simulink model "Main_simulation_optimised_accel_testbed"  (R2017b)
settings: Solver=FixedStepDiscrete  StartTime=0  StopTime=2474  RelTol=1e-3  EnableMultiTasking=on
PreLoadFcn:
  | Ts=2e-6;
undefined symbols (not defined in the file): Batt, BatteryCback, BatteryLoadFcn, DiscIntNeverNeededParam, Discrete, gcbh, Ion, Lithium, sigbuilder_block, sps_rtmsupport, spsBatteryModel
libraries: powerlib x53, electricdrivelib x6, simulink x6, autolibshared x6, powerlib_meascontrol x4, sdolib x3, spsDrivesDcBusModel x1, spsDrivesPrivateModels x1, spsDrivesOutputSelector x1, spsDrivesSpeedControllerModel x1
(part 1 of 3)
Description:
  | Copyright 2008-2017 The MathWorks, Inc.
settings Model: SimulationMode=accelerator  ExtModeAutoUpdateStatusClock=off  Creator=MathWorks  LastModifiedBy=LENOVO
settings SolverCC: AlgebraicLoopSolver=LineSearch  AutoInsertRateTranBlk=on
settings DataIOCC: LimitDataPoints=on  SaveFormat=Array  SignalLoggingSaveFormat=ModelDataLogs  SaveOutput=off  SignalLogging=off  SaveTime=off  SignalLoggingName=sigsOut
settings OptimizationCC: ExpressionDepthLimit=2147483647  InitFltsAndDblsToZero=on  LifeSpan=inf
settings DebuggingCC: UnderspecifiedInitializationDetection=Classic  MergeDetectMultiDrivingBlocksExec=none  CheckExecutionContextPreStartOutputMsg=on  CheckExecutionContextRuntimeOutputMsg=on  SignalResolutionControl=TryResolveAllWithWarning  MultiTaskDSMMsg=warning  MultiTaskCondExecSysMsg=none  FcnCallInpInsideContextMsg=warning  StateNameClashWarn=warning  SFUnexpectedBacktrackingDiag=warning  SFNoUnconditionalDefaultTransitionDiag=warning  SFExecutionAtInitializationDiag=none
settings HardwareCC: ProdBitPerPointer=32  ProdBitPerSizeT=32  ProdBitPerPtrDiffT=32  ProdLargestAtomicFloat=None  ProdIntDivRoundTo=Undefined  ProdEndianess=Unspecified  ProdWordSize=32  ProdHWDeviceType=32-bit Generic  TargetUnknown=on
settings ModelReferenceCC: PropagateSignalLabelsOutOfModel=off
settings CodeAppCC: StateflowObjectComments=on
settings GRTTargetCC: TargetLangStandard=C89/C90 (ANSI)  GeneratePreprocessorConditionals=Disable all  CombineOutputUpdateFcns=off  GRTInterface=on
settings ConfigComp: CovMetricSettings=dw  CovHtmlReporting=on  CovSaveCumulativeToWorkspaceVar=on  CovSaveSingleToWorkspaceVar=on  CovExternalEMLEnable=off  CovSFcnEnable=off
settings SimscapeCC: SimscapeNormalizeSystem=off

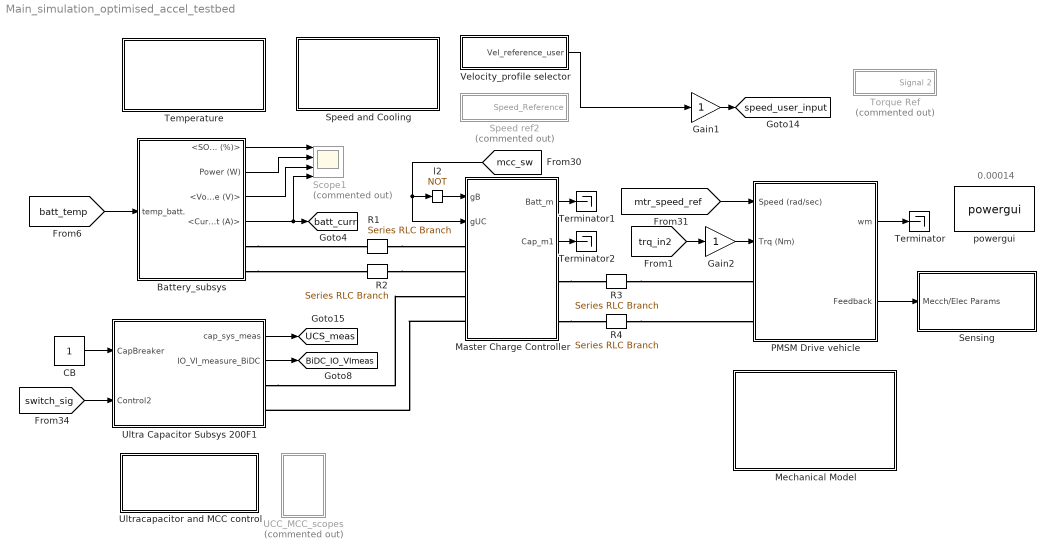
== system Main_simulation_optimised_accel_testbed ==
  note: 0.00014
  Battery_subsys : Subsystem
  CB : Constant
  Gain1 : Gain
  Gain2 : Gain
  Master Charge Controller : Subsystem
  Mechanical Model : Subsystem
  PMSM Drive vehicle : Subsystem
  R{1..4} (4 alike) : powerlib/Elements/Series RLC Branch  LConnTagsString=__new0  RConnTagsString=__new0  BranchType=R  Resistance=0.02  Inductance=220e-6  SetiL0=off  InitialCurrent=0  Capacitance=447e-6  Setx0=off  InitialVoltage=0  Measurements=None
  Scope1 : Scope  Commented=on  NumInputPorts=4
  Sensing : Subsystem
  "Speed and Cooling " : Subsystem
  Speed ref2 : Subsystem  Tag=STV Subsys  Commented=on  LoadFcn=sigbuilder_block('load');  StartFcn=sigbuilder_block('start');  StopFcn=sigbuilder_block('stop');  ClipboardFcn=sigbuilder_block('clipboard');  mask(Sigbuilder block){tuvar=[0:10]}
      mask help: Simulink:masks:SigbuilderBlock_MD
      mask init:
      | if ~strcmp(get_param(bdroot(gcbh),'SimulationStatus'),'stopped') tuvar = sigbuilder_block('maskInit'); end
      settings: CopyFcn=sigbuilder_block('copy');  DeleteFcn=sigbuilder_block('delete');  ModelCloseFcn=sigbuilder_block('modelClose');  PreSaveFcn=sigbuilder_block('preSave');  PauseFcn=sigbuilder_block('pause');  ContinueFcn=sigbuilder_block('continue');  NameChangeFcn=sigbuilder_block('namechange');  OpenFcn=sigbuilder_block('open',[5.4 30 1141.2 522.6 ]);  CloseFcn=sigbuilder_block('close');
      mask Display: plot(0, 0, 100, 100,[2, 2, 32, 32, 2], [68, 8, 8, 68, 68],[32, 2], [38, 38], [32, 19, 2],[53, 60, 44], [32, 17, 17, 2],[16, 16, 31, 31]);txt = getActiveGroup(gcbh);text(2, 100, txt,'verticalAlignment', 'top');
  Temperature : Subsystem
  Terminator : Terminator
  Terminator1 : Terminator
  Terminator2 : Terminator
  Torque Ref : Subsystem  Tag=STV Subsys  Commented=on  LoadFcn=sigbuilder_block('load');  StartFcn=sigbuilder_block('start');  StopFcn=sigbuilder_block('stop');  ClipboardFcn=sigbuilder_block('clipboard');  mask(Sigbuilder block){tuvar=[0:10]}
      mask help: Simulink:masks:SigbuilderBlock_MD
      mask init:
      | if ~strcmp(get_param(bdroot(gcbh),'SimulationStatus'),'stopped') tuvar = sigbuilder_block('maskInit'); end
      settings: CopyFcn=sigbuilder_block('copy');  DeleteFcn=sigbuilder_block('delete');  ModelCloseFcn=sigbuilder_block('modelClose');  PreSaveFcn=sigbuilder_block('preSave');  PauseFcn=sigbuilder_block('pause');  ContinueFcn=sigbuilder_block('continue');  NameChangeFcn=sigbuilder_block('namechange');  OpenFcn=sigbuilder_block('open',[5.4 30 1141.2 522.6 ]);  CloseFcn=sigbuilder_block('close');
      mask Display: plot(0, 0, 100, 100,[2, 2, 32, 32, 2], [68, 8, 8, 68, 68],[32, 2], [38, 38], [32, 19, 2],[53, 60, 44], [32, 17, 17, 2],[16, 16, 31, 31]);txt = getActiveGroup(gcbh);text(2, 100, txt,'verticalAlignment', 'top');
  "UCC_MCC_scopes " : Subsystem  Commented=on
  Ultra Capacitor Subsys 200F1 : Subsystem
  Ultracapacitor and MCC control : Subsystem
  Velocity_profile selector : Subsystem
  l2 : Logic  Operator=NOT  IconShape=distinctive  AllPortsSameDT=off  OutDataTypeStr=boolean
  powergui : powerlib/powergui  Priority=2  SimulationMode=Discrete  SampleTime=1e-6  frequency=60  Iterations=50  frequencyindice=0  Pbase=100e6  ErrMax=1e-4  UnitsV=kV  UnitsW=MW  buscounter=0  FunctionMessages=off  echomessages=off  EnableUseOfTLC=off  CurrentSourceSwitches=off  DisableSnubberDevices=off  DisableRonSwitches=off  DisableVfSwitches=off  DisplayEquations=off  SolverType=Tustin/Backward Euler (TBE)  Interpol=off  ExternalGateDelay=off  methode=off  Ts=0  x0status=blocks  SPID=off  SwTol=0  HookPort=off  RestoreLinks=warning  ResistiveCurrentMeasurement=off  Frange=[0:2:500]  Ylog=off  Xlog=on  ShowGrid=off  save=off  variable=ZData  structure=0  ZoomFFT=on  StartTime=0.0  cycles=1  DisplayStyle=1  fundamental=60  FreqAxis=off  MaxFrequency=1000  frequencyindicesteady=1  RmsSteady=1  display=off
  tag scope: BiDC_IO_VImeas=global, UCS_meas=global, batt_curr=global, speed_user_input=global
  wires:
  Velocity_profile selector/1(Vel_reference_user) -> Gain1/1
  [trq_in2] -> Gain2/1
  Gain2/1 -> PMSM Drive vehicle/2(Trq (Nm))
  PMSM Drive vehicle/1(wm) -> Terminator/1
  PMSM Drive vehicle/2(Feedback) -> Sensing/1(Mecch/Elec Params)
  Battery_subsys/4(<Current (A)>) -> Scope1/4, [batt_curr]
  [batt_temp] -> Battery_subsys/1(temp_batt.)
  Battery_subsys/2(Power (W)) -> Scope1/2
  Battery_subsys/1(<SOC (%)>) -> Scope1/1
  Battery_subsys/3(<Voltage (V)>) -> Scope1/3
  [mcc_sw] -> Master Charge Controller/2(gUC), l2/1
  CB/1 -> Ultra Capacitor Subsys 200F1/1(CapBreaker)
  Ultra Capacitor Subsys 200F1/1(cap_sys_meas) -> [UCS_meas]
  l2/1 -> Master Charge Controller/1(gB)
  [switch_sig] -> Ultra Capacitor Subsys 200F1/2(Control2)
  [mtr_speed_ref] -> PMSM Drive vehicle/1(Speed (rad/sec))
  Ultra Capacitor Subsys 200F1/2(IO_VI_measure_BiDC) -> [BiDC_IO_VImeas]
  Master Charge Controller/1(Batt_m) -> Terminator1/1
  Master Charge Controller/2(Cap_m1) -> Terminator2/1
  Gain1/1 -> [speed_user_input]
  connections:
  Master Charge Controller/RConn1 -- R3/RConn1
  Master Charge Controller/RConn2 -- R4/RConn1
  Battery_subsys/RConn1 -- R1/RConn1
  Battery_subsys/RConn2 -- R2/RConn1
  Ultra Capacitor Subsys 200F1/RConn1 -- Master Charge Controller/LConn3
  Master Charge Controller/LConn4 -- Ultra Capacitor Subsys 200F1/RConn2
  R1/LConn1 -- Master Charge Controller/LConn1
  R2/LConn1 -- Master Charge Controller/LConn2
  R3/LConn1 -- PMSM Drive vehicle/LConn1
  R4/LConn1 -- PMSM Drive vehicle/LConn2

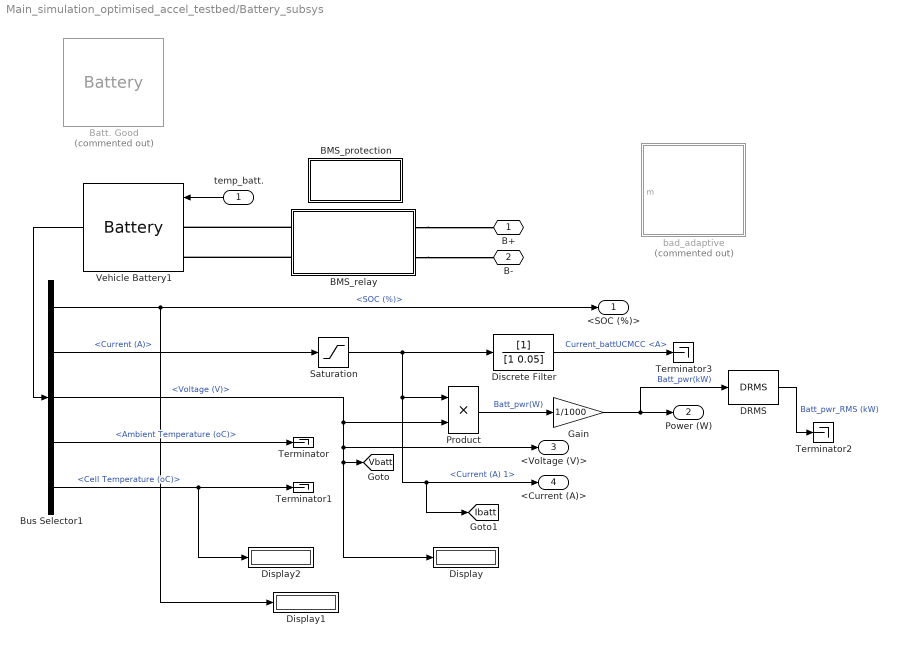
== system Main_simulation_optimised_accel_testbed/Battery_subsys ==
  temp_batt. : Inport
  BMS_protection : Subsystem
  BMS_relay : Subsystem
  Batt. Good : electricdrivelib/Extra Sources/Battery  Commented=on  BatType=Lithium-Ion  ShowTempParam=on  ThermalPreset=no  ShowAgeParam=off  NomV=120  NomQ=66  SOC=96  Batt_Tr=0.1  PresetModel=off  MaxQ=66  MinV=90  FullV=130  Dis_rate=30  R=0.018182  Normal_OP=59.687  expZone="[129.6463      3.242609]"  current=[6.5 13 18 22 32.5 40]  Units=Time  Tci=20  NomT=50  T2=-15  MaxQ2=60*0.7  FullV2=117  Normal_OP2=120*0.9  expZone2="[120        50]"  Rca=0.5  ti=1  Dp=0  Neq0=1  Tsim=50e-6  Ta1=35  Qeol=60*0.85  Reol=0.013333*1.2  Char_age=[2.3478, 3]  Dis_age=[2.3478, 10]  N1=1500  N2=10500  N3=1000  N4=1400  Ta2=45  N5=950
  Bus Selector1 : BusSelector  OutputSignals=SOC (%),Current (A),Voltage (V),Ambient Temperature (oC),Cell Temperature (oC)
  DRMS : sdolib/RMS Blocks/DRMS  Ts=10e-6
      settings: SourceProductName=Simulink Design Optimization  SourceProductBaseCode=SO
  Discrete Filter : DiscreteFilter  Denominator=[1 0.05]
  Display : Display
  Display1 : Display
  Display2 : Display
  Gain : Gain  Gain=1/1000
  Product : Product
  Saturation : Saturate  UpperLimit=50  LowerLimit=-40
  Terminator{,1..3} (4 alike) : Terminator
  Vehicle Battery1 : electricdrivelib/Extra Sources/Battery  BatType=Lithium-Ion  ShowTempParam=on  ThermalPreset=no  ShowAgeParam=off  NomV=120  NomQ=66  SOC=30  Batt_Tr=0.1  PresetModel=off  MaxQ=66  MinV=90  FullV=130  Dis_rate=30  R=0.018182  Normal_OP=59.687  expZone="[129.6463      3.242609]"  current=[6.5 13 18 22 32.5 40]  Units=Time  Tci=20  NomT=50  T2=-15  MaxQ2=60*0.7  FullV2=117  Normal_OP2=120*0.9  expZone2="[120        50]"  Rca=0.5  ti=1  Dp=0  Neq0=1  Tsim=50e-6  Ta1=35  Qeol=60*0.85  Reol=0.013333*1.2  Char_age=[2.3478, 3]  Dis_age=[2.3478, 10]  N1=1500  N2=10500  N3=1000  N4=1400  Ta2=45  N5=950
  bad_adaptive : Subsystem  Commented=on  DialogController=POWERSYS.PowerSysDialog  LoadFcn=sps_rtmsupport('LoadFcn',gcbh); BatteryLoadFcn(gcb)  InitFcn=BatteryCback(gcb,1)  StartFcn=sps_rtmsupport('StartFcn',gcbh);  StopFcn=sps_rtmsupport('StopFcn',gcbh);  mask(Battery){BatType=Lithium-Ion, ShowTempParam=off, ThermalPreset=no, ShowAgeParam=off, NomV=120, NomQ=66, SOC=96, Batt_Tr=0.1, PresetModel=off, MaxQ=66, MinV=90, FullV=130, Dis_rate=30, R=0.018182, Normal_OP=59.687, expZone=[129.6463      3.242609], current=[6.5 13 18 22 32.5 40], Units=Time, Tci=20, NomT=50, T2=-15, MaxQ2=60*0.7, FullV2=117, Normal_OP2=120*0.9, expZone2=[120        50], Rca=0.5, ti=1, Dp=0, Neq0=1, Tsim=50e-6, Ta1=35, Qeol=60*0.85, Reol=0.013333*1.2, Char_age=[2.3478, 3], Dis_age=[2.3478, 10], N1=1500, N2=10500, N3=1000, N4=1400, Ta2=45, N5=950}
      mask prompts: BatType "Type:"; ShowTempParam "Simulate temperature effects"; ThermalPreset "Use a preset battery:"; ShowAgeParam "Simulate aging effects"; NomV "Nominal voltage (V)"; NomQ "Rated capacity (Ah)"; SOC "Initial state-of-charge (%)"; Batt_Tr "Battery response time (s)"; PresetModel "Determined from the nominal parameters of the battery"; MaxQ "Maximum capacity (Ah)"; MinV "Cut-off Voltage (V)"; FullV "Fully charged voltage (V)"; Dis_rate "Nominal discharge current (A)"; R "Internal resistance (Ohms)"; Normal_OP "Capacity (Ah) at nominal voltage"; expZone "Exponential zone [Voltage (V), Capacity (Ah)]"; current "Discharge current [i1, i2, i3,...] (A)"; Tci "Initial cell temperature (deg. C)"; NomT "Nominal ambient temperature T1 (deg. C)"; T2 "Second ambient temperature T2 (deg. C)"; MaxQ2 "Maximum capacity (Ah)"; FullV2 "Initial discharge voltage (V)"; Normal_OP2 "Voltage at 90% maximum capacity (V)"; expZone2 "Exponential zone [Voltage (V), Capacity (Ah)]"; Rca "Thermal resistance, cell-to-ambient (deg. C/W)"; ti "Thermal time constant, cell-to-ambient (s)"; Dp "Heat loss difference [charge vs. discharge] (W)"; Neq0 "Initial battery age (Equivalent full cycles)"; Tsim "Aging model sampling time (s)"; Ta1 "Ambient temperature Ta1 (deg. C)"; Qeol "Capacity at EOL (End Of Life) (Ah)"; Reol "Internal resistance at EOL (Ohms)"; Char_age "Charge current (nominal, maximum) [Ic (A), Icmax (A)]"; Dis_age "Discharge current (nominal, maximum) [Id (A), Idmax (A)]"; N1 "Cycle life at 100 % DOD, Ic and Id (Cycles)"; N2 "Cycle life at 25 % DOD, Ic and Id (Cycles)"; N3 "Cycle life at 100 % DOD, Ic and Idmax (Cycles)"; N4 "Cycle life at 100 % DOD, Icmax and Id (Cycles)"; Ta2 "Ambient temperature Ta2 (deg. C)"; N5 "Cycle life at 100 % DOD, Ic and Id (Cycles)"
      mask help: Implements a generic battery model for most popular battery types. Temperature and aging (due to cycling) effects can be specified for Lithium-Ion battery type.
      mask init:
      | block = gcb;
      | BatteryCback(block,3)
      | [Batt BT, WantBlockChoice, Ts] = BatteryParam(NomV,NomQ,MaxQ,MinV,FullV,Dis_rate,R,Normal_OP,expZone,block,0);
      | powericon('SetInternalModels','set',block,WantBlockChoice);
      | BatteryCback(block,1);
      settings: CopyFcn=sps_rtmsupport('CopyFcn',gcbh);  DeleteFcn=sps_rtmsupport('DeleteFcn',gcbh);  UndoDeleteFcn=sps_rtmsupport('UndoDeleteFcn',gcbh);  ModelCloseFcn=sps_rtmsupport('ModelCloseFcn',gcbh);  PreSaveFcn=sps_rtmsupport('PreSaveFcn',gcbh);  PostSaveFcn=sps_rtmsupport('PostSaveFcn',gcbh);  NameChangeFcn=sps_rtmsupport('NameChangeFcn',gcbh);  PreCopyFcn=sps_rtmsupport('PreCopyFcn',gcbh);  OpenFcn=sps_rtmsupport('OpenFcn',gcbh, [1,2,3,4,9,18]);  CloseFcn=sps_rtmsupport('CloseFcn',gcbh);  PreDeleteFcn=sps_rtmsupport('PreDeleteFcn',gcbh);
      mask Help: helpview(psbhelp)
      mask TypeOptions BatType: Lead-Acid | Lithium-Ion | Nickel-Cadmium | Nickel-Metal-Hydride
      mask Callback BatType: BatteryCback(gcb,1)
      mask Callback ShowTempParam: BatteryCback(gcb,1)
      mask TypeOptions ThermalPreset: no | 3.3V  2.3Ah  (LiFePO4) | 3.6V  2050mAh   (LiCoO2) | 3.6V  2.0Ah | 3.6V  3.6Ah  (LiNiO2) | 3.6V  4.5Ah | 3.6V  48Ah  (LiNiO2) | 3.7V  4.4Ah | 7.4V  5.4Ah  (LiCoO2) | 11.1V  6600mAh  (LiCoO2) | 12.8V  40Ah  (LiFeMgPO4)
      mask Callback ThermalPreset: BatteryCback(gcb,4)
      mask Callback ShowAgeParam: BatteryCback(gcb,1)
      mask Callback PresetModel: BatteryCback(gcb,1)
      mask TypeOptions Units: Ampere-hour | Time
      mask Callback ti: sps_rtmsupport('parametereditingmodes',gcbh, [1,2,3,4,9,18]);
      mask DialogControl ParameterTabVar0 Prompt: Parameters
      mask DialogControl Tempcontainer Prompt: Temperature
      mask DialogControl Agecontainer Prompt: Aging
      mask DialogControl ParameterTabVar01 Prompt: Discharge
      mask DialogControl Container9 Prompt: Display characteristics
      mask DialogControl PlotButton Prompt: Plot
      mask DialogControl PlotButton Callback: BatteryCback(gcb,0)
      mask DialogControl Temperature Prompt: Temperature
      mask DialogControl Container7 Prompt: Discharge parameters at T2
      mask DialogControl Container8 Prompt: Thermal response and Heat loss
      mask DialogControl Aging Prompt: Aging
      mask DialogControl Container16 Prompt: Aging characteristics at ambient temperature Ta1
      mask DialogControl Container13 Prompt: Aging characteristics at ambient temperature Ta2
      mask Display:
      | patch([BT.X1 BT.X1m],[BT.Y1 BT.Y1m],BT.color1);
      | patch(BT.X3,BT.Y3,BT.color2);
      | plot([BT.X1 BT.X1m BT.X2 BT.X2m BT.X3 BT.X4],[BT.Y1 BT.Y1m BT.Y2 BT.Y2m BT.Y3 BT.Y4]);
      | plot(-100,-60,60,50,[BT.X(1) BT.X(1)],[BT.bas BT.haut],[BT.X(2) BT.X(2)],[BT.haut BT.bas],BT.dim_Xsin,4*sin(BT.dim_sin)+BT.haut,BT.dim_Xsin,-4*sin(BT.dim_sin)+BT.haut,BT.dim_Xsin,-4*sin(BT.dim_sin)+BT.bas,BT.dim_Xtop,sin(BT.dim_top)+BT.haut+4,BT.dim_Xtop,-sin(BT.dim_top)+BT.haut+4,BT.dim_Xtop,-sin(BT.dim_top)+BT.haut,[BT.TopX(2),BT.TopX(2)],[BT.haut,BT.haut+4],[BT.TopX(1),BT.TopX(1)],[BT.haut+4,BT.haut]);plot(BT.dim_Xsin,-5*sin(BT.dim_sin)+20);
      | port_label('lconn',1,'+');
      | port_label('lconn',2,'_');
      | color('blue');
      | port_label('output',1,'m');
      | 
      | if Batt.sel_T
      |     port_label('input',1,'Ta');
      | end
  B+ : PMIOPort  Port=1  Side=Right
  B- : PMIOPort  Port=2  Side=Right
  <SOC (%)> : Outport
  Power (W) : Outport  Port=2
  <Voltage (V)> : Outport  Port=3
  <Current (A)> : Outport  Port=4
  tag scope: Ibatt=global, Vbatt=global
  wires:
  temp_batt./1 -> Vehicle Battery1/1
  Bus Selector1/2 -> Saturation/1  "<Current (A)>"
  Bus Selector1/1 -> Display1/1, <SOC (%)>/1  "<SOC (%)>"
  Product/1 -> Gain/1  "Batt_pwr(W)"
  Vehicle Battery1/1 -> Bus Selector1/1
  Bus Selector1/3 -> Product/2, <Voltage (V)>/1, Display/1, [Vbatt]  "<Voltage (V)>"
  Gain/1 -> Power (W)/1, DRMS/1  "Batt_pwr(kW)"
  Saturation/1 -> Product/1, <Current (A)>/1, [Ibatt], Discrete Filter/1  "<Current (A) 1>"
  Bus Selector1/4 -> Terminator/1  "<Ambient Temperature (oC)>"
  Bus Selector1/5 -> Display2/1, Terminator1/1  "<Cell Temperature (oC)>"
  DRMS/1 -> Terminator2/1  "Batt_pwr_RMS (kW)"
  Discrete Filter/1 -> Terminator3/1  "Current_battUCMCC <A>"
  connections:
  BMS_relay/LConn1 -- Vehicle Battery1/LConn1
  BMS_relay/LConn2 -- Vehicle Battery1/LConn2
  BMS_relay/RConn1 -- B+/RConn1
  BMS_relay/RConn2 -- B-/RConn1

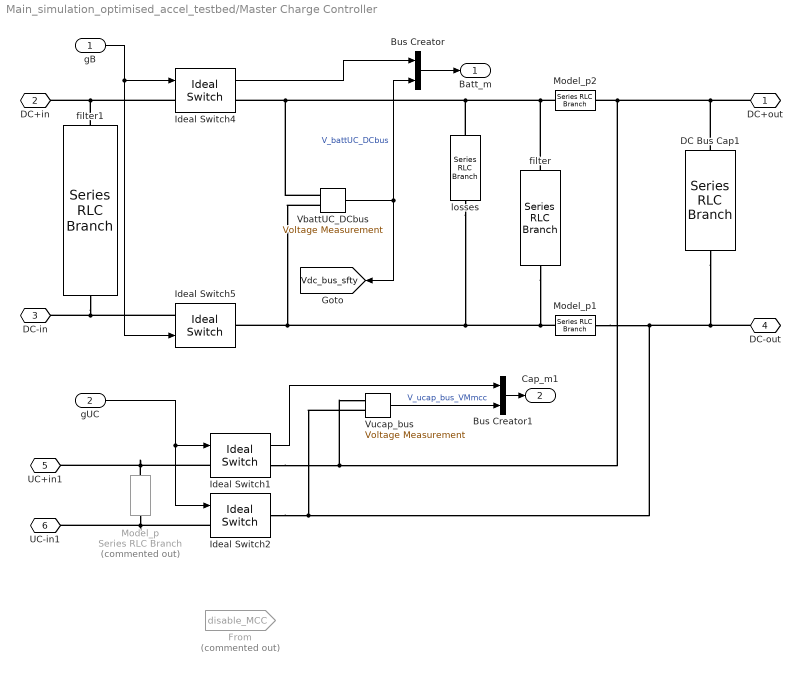
== system Main_simulation_optimised_accel_testbed/Master Charge Controller ==
  gB : Inport
  gUC : Inport  Port=2
  Bus Creator : BusCreator  Inputs=2
  Bus Creator1 : BusCreator  Inputs=2
  DC Bus Cap1 : powerlib/Elements/Series RLC Branch  LConnTagsString=__new0  RConnTagsString=__new0  BranchType=RC  Resistance=1e-2  Inductance=1e-3  SetiL0=off  InitialCurrent=0  Capacitance=400e-6  Setx0=off  InitialVoltage=0  Measurements=None
  From : From  Commented=on  GotoTag=disable_MCC  TagVisibility=global
  Ideal Switch1 : powerlib/Power Electronics/Ideal Switch  Ron=0.001  Lon=0  IC=0  Rs=1e6  Cs=10e-6  Measurements=on
  Ideal Switch2 : powerlib/Power Electronics/Ideal Switch  Ron=0.001  Lon=0  IC=0  Rs=1e6  Cs=10e-6  Measurements=off
  Ideal Switch4 : powerlib/Power Electronics/Ideal Switch  Ron=0.001  Lon=0  IC=0  Rs=10e6  Cs=10e-6  Measurements=on
  Ideal Switch5 : powerlib/Power Electronics/Ideal Switch  Ron=0.001  Lon=0  IC=0  Rs=10e6  Cs=10e-6  Measurements=off
  Model_p : powerlib/Elements/Series RLC Branch  Commented=on  LConnTagsString=__new0  RConnTagsString=__new0  BranchType=R  Resistance=10e6  Inductance=1e-3  SetiL0=off  InitialCurrent=0  Capacitance=0  Setx0=off  InitialVoltage=0  Measurements=None
  Model_p1 : powerlib/Elements/Series RLC Branch  LConnTagsString=__new0  RConnTagsString=__new0  BranchType=RL  Resistance=0.01  Inductance=20e-6  SetiL0=off  InitialCurrent=0  Capacitance=0  Setx0=off  InitialVoltage=0  Measurements=None
  Model_p2 : powerlib/Elements/Series RLC Branch  LConnTagsString=__new0  RConnTagsString=__new0  BranchType=RL  Resistance=0.01  Inductance=20e-6  SetiL0=off  InitialCurrent=0  Capacitance=0  Setx0=off  InitialVoltage=0  Measurements=None
  VbattUC_DCbus : powerlib/Measurements/Voltage Measurement  PhasorSimulation=off  OutputType=Complex  PSBequivalent=0
  Vucap_bus : powerlib/Measurements/Voltage Measurement  PhasorSimulation=off  OutputType=Complex  PSBequivalent=0
  filter : powerlib/Elements/Series RLC Branch  LConnTagsString=__new0  RConnTagsString=__new0  BranchType=RC  Resistance=1e-3  Inductance=1e-3  SetiL0=off  InitialCurrent=0  Capacitance=1e-6  Setx0=off  InitialVoltage=0  Measurements=None
  filter1 : powerlib/Elements/Series RLC Branch  LConnTagsString=__new0  RConnTagsString=__new0  BranchType=RC  Resistance=1e-3  Inductance=1e-3  SetiL0=off  InitialCurrent=0  Capacitance=1e-6  Setx0=off  InitialVoltage=0  Measurements=None
  losses : powerlib/Elements/Series RLC Branch  LConnTagsString=__new0  RConnTagsString=__new0  BranchType=R  Resistance=10e6  Inductance=1e-3  SetiL0=off  InitialCurrent=0  Capacitance=1e-6  Setx0=off  InitialVoltage=0  Measurements=None
  DC+out : PMIOPort  Port=1  Side=Right
  DC+in : PMIOPort  Port=2  Side=Left
  DC-in : PMIOPort  Port=3  Side=Left
  DC-out : PMIOPort  Port=4  Side=Right
  UC+in1 : PMIOPort  Port=5  Side=Left
  UC-in1 : PMIOPort  Port=6  Side=Left
  Batt_m : Outport
  Cap_m1 : Outport  Port=2
  tag scope: Vdc_bus_sfty=global
  wires:
  gB/1 -> Ideal Switch5/1, Ideal Switch4/1
  Ideal Switch4/1 -> Bus Creator/1
  Ideal Switch1/1 -> Bus Creator1/1
  gUC/1 -> Ideal Switch2/1, Ideal Switch1/1
  VbattUC_DCbus/1 -> [Vdc_bus_sfty], Bus Creator/2  "V_battUC_DCbus"
  Bus Creator/1 -> Batt_m/1
  Bus Creator1/1 -> Cap_m1/1
  Vucap_bus/1 -> Bus Creator1/2  "V_ucap_bus_VMmcc"
  connections:
  Vucap_bus/LConn2 -- Ideal Switch2/RConn1 -- DC-out/RConn1 -- DC Bus Cap1/RConn1 -- Model_p1/LConn1
  Vucap_bus/LConn1 -- Ideal Switch1/RConn1 -- DC+out/RConn1 -- DC Bus Cap1/LConn1 -- Model_p2/LConn1
  Ideal Switch4/LConn1 -- filter1/LConn1 -- DC+in/RConn1
  Ideal Switch5/LConn1 -- filter1/RConn1 -- DC-in/RConn1
  Ideal Switch1/LConn1 -- Model_p/LConn1 -- UC+in1/RConn1
  Ideal Switch2/LConn1 -- Model_p/RConn1 -- UC-in1/RConn1
  losses/RConn1 -- VbattUC_DCbus/LConn2 -- Ideal Switch5/RConn1 -- Model_p1/RConn1 -- filter/RConn1
  losses/LConn1 -- Model_p2/RConn1 -- filter/LConn1 -- VbattUC_DCbus/LConn1 -- Ideal Switch4/RConn1

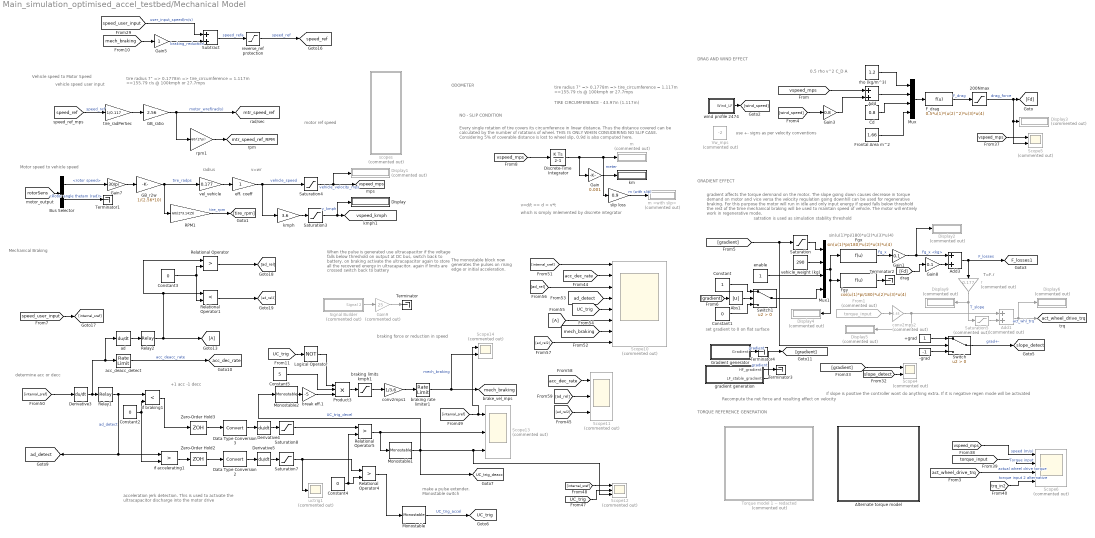
== system Main_simulation_optimised_accel_testbed/Mechanical Model ==
  note: sin(u(1)*pi/180)*u(2)*u(3)*u(4)
  note: set gradient to 0 on flat surface
  note: Recompute the net force and resulting effect on velocity
  note: Vehicle speed to Motor Speed
  note: motor ref speed
  note: tire radius 7" => 0.1778m => tire_circumference = 1.117m
      | =>155.79 r/s @ 100kmph or 27.7mps
  note: vehicle speed
      | user input
  note: v=wr
  note: Motor speed to vehicle speed
  note: radius
  note: T=F.r
  note: use +- signs as per velocity conventions
  note: satration is used as simulation stability threshold
  note: gradient affects the torque demnand on the motor. The slope going down causes decrease in torque demand on motor and vice versa
      |
      | the velocity regulation going downhill can be used for regenerative braking. For this purpose the motor will run in idle and only input energy if speed falls below threshold
      | the rest of the time mechanical braking will be used to maintain speed of vehicle. The motor will entirely work in regenerative mode.
  note: if slope is positive the controller wont do anything extra. If it is negative regen mode will be activated
  note: 0.5 rho v^2 C_D A
  note: GRADIENT EFFECT
  note: DRAG AND WIND EFFECT
  note: TORQUE REFERENCE GENERATION
  note: make a pulse extender.
      | Monostable switch
  note: acceleration jerk detection. This is used to activate the ultracapacitor discharge into the motor drive
  note: When the pulse is generated use ultracapacitor
      | if the voltage falls below threshold on output
      | at DC bus, switch back to battery.
      |
      | on braking activate the ultracapacitor again to store all
      | the recovered energy in ultracapacitor. again if limits are
      | crossed switch back to battery
  note: The monostable block
      | now generates the
      | pulses on rising edge or
      | initial acceleration.
  note: Mechanical Braking
  note: braking force or reduction in speed
  note: determine acc or decc
  note: +1 acc
      |  -1 decc
  note: NO - SLIP CONDITION
  note: which is simply imlemented by discrete integrator
  note: v=d/t => d = v*t
  note: ODOMETER
  note: Every single rotation of tire covers its circumference in linear distance. Thus the distance covered
      | can be calculated by the number of rotations of wheel. THIS IS ONLY WHEN CONSIDERING
      | NO SLIP CASE. Considering 5% of coverable distance is lost to wheel slip, 0.9d is also computed here.
  note: TIRE CIRCUMFERENCE - 43.97in (1.117m)
  note: tire radius 7" => 0.1778m => tire_circumference = 1.117m
      | =>155.79 r/s @ 100kmph or 27.7mps
  +grad : Constant
  -grad : Constant  Value=-1
  200Nmax : Saturate  UpperLimit=200  LowerLimit=0
  Abs1 : Abs
  Add : Sum
  Add1 : Sum  Commented=on
  Add3 : Sum
  Alternate torque model : Subsystem
  Bus Selector : BusSelector  OutputSignals=rotor speed,Rotor angle thetam (rad)
  Cd : Constant  Value=0.8
  Constant : Constant
  Constant{1..4} (4 alike) : Constant  Value=0
  Constant5 : Constant  Value=5
  Data Type Conversion2 : DataTypeConversion
  Data Type Conversion3 : DataTypeConversion
  Derivative3 : Derivative
  Derivative4 : Derivative
  Derivative5 : Derivative
  Discrete-Time Integrator : DiscreteIntegrator  InitialConditionSetting=State (most efficient)  SampleTime=-1  ICPrevOutput=DiscIntNeverNeededParam  ICPrevScaledInput=DiscIntNeverNeededParam
  Display : Display
  Display{1..6,9} (7 alike) : Display  Commented=on
  F_drag : Fcn  Expr=0.5*u(1)*(u(2)^2)*u(3)*u(4)
  Fgx : Fcn  Expr=sin(u(1)*pi/180)*u(2)*u(3)*u(4)
  Fgy : Fcn  Expr=cos(u(1)*pi/180)*u(2)*u(3)*u(4)
  From1 : From  Commented=on  GotoTag=torque_input  TagVisibility=global
  Frontal Area m^2 : Constant  Value=1.66
  GB_r2w : Gain  Gain=1/(2.56*10)
  GB_ratio : Gain  Gain=2.56
  Gain : Gain  Gain=0.001
  Gain1 : Gain  Gain=0.1
  Gain3 : Gain  Gain=0.8
  Gain5 : Gain
  Gain7 : Gain  Gain=30/pi  SaturateOnIntegerOverflow=on  OutDataTypeStr=Inherit: Same as input  ParamDataTypeStr=Inherit: Same as input
  Gain8 : Gain  Gain=0.1
  Gain9 : Gain  Commented=on  Gain=25
  Gradient generator : Subsystem  Tag=STV Subsys  LoadFcn=sigbuilder_block('load');  StartFcn=sigbuilder_block('start');  StopFcn=sigbuilder_block('stop');  ClipboardFcn=sigbuilder_block('clipboard');  mask(Sigbuilder block){tuvar=[0:10]}
      mask help: Simulink:masks:SigbuilderBlock_MD
      mask init:
      | if ~strcmp(get_param(bdroot(gcbh),'SimulationStatus'),'stopped') tuvar = sigbuilder_block('maskInit'); end
      settings: CopyFcn=sigbuilder_block('copy');  DeleteFcn=sigbuilder_block('delete');  ModelCloseFcn=sigbuilder_block('modelClose');  PreSaveFcn=sigbuilder_block('preSave');  PauseFcn=sigbuilder_block('pause');  ContinueFcn=sigbuilder_block('continue');  NameChangeFcn=sigbuilder_block('namechange');  OpenFcn=sigbuilder_block('open',[0 30 1152 561.6 ]);  CloseFcn=sigbuilder_block('close');
      mask Display: plot(0, 0, 100, 100,[2, 2, 32, 32, 2], [68, 8, 8, 68, 68],[32, 2], [38, 38], [32, 19, 2],[53, 60, 44], [32, 17, 17, 2],[16, 16, 31, 31]);txt = getActiveGroup(gcbh);text(2, 100, txt,'verticalAlignment', 'top');
  Logical Operator : Logic  Operator=NOT  IconShape=distinctive  AllPortsSameDT=off  OutDataTypeStr=boolean
  Monostable : powerlib_meascontrol/Logic/Monostable  EdgeDetect=Rising  PulseDuration=0.4  ic=0  Ts=0
      settings: SourceProductName=Simscape Power Systems  SourceProductBaseCode=PS
  Monostable1 : powerlib_meascontrol/Logic/Monostable  EdgeDetect=Rising  PulseDuration=0.15  ic=0  Ts=0
      settings: SourceProductName=Simscape Power Systems  SourceProductBaseCode=PS
  Monostable2 : powerlib_meascontrol/Logic/Monostable  EdgeDetect=Rising  PulseDuration=0.45  ic=0  Ts=0
      settings: SourceProductName=Simscape Power Systems  SourceProductBaseCode=PS
  Mux : Mux
  Mux1 : Mux
  Product3 : Product  Inputs=3
  RPM1 : Gain  Gain=60/(2*3.1415)
  Relational Operator : RelationalOperator  Operator=>  OutDataTypeStr=boolean  RndMeth=Simplest
  Relational Operator1 : RelationalOperator  Operator=<  OutDataTypeStr=boolean  RndMeth=Simplest
  Relational Operator4 : RelationalOperator  Operator=>  OutDataTypeStr=boolean  RndMeth=Simplest
  Relational Operator5 : RelationalOperator  Operator=>  OutDataTypeStr=boolean  RndMeth=Simplest
  Relay1 : Relay  OffOutputValue=-1
  Relay2 : Relay  OffOutputValue=-1
  Saturation : Saturate  UpperLimit=10  LowerLimit=-10
  Saturation3 : Saturate  UpperLimit=108  LowerLimit=0
  Saturation4 : Saturate  UpperLimit=30  LowerLimit=0
  Saturation5 : Saturate  Commented=on  UpperLimit=25  LowerLimit=-25
  Saturation7 : Saturate  UpperLimit=10  LowerLimit=-10
  Saturation8 : Saturate  UpperLimit=10  LowerLimit=-10
  Scope10 : Scope  Commented=on  NumInputPorts=8
  Scope11 : Scope  Commented=on  NumInputPorts=3
  Scope12 : Scope  Commented=on  NumInputPorts=3
  Scope13 : Scope  Commented=on  NumInputPorts=3
  Scope14 : Scope  Commented=on  NumInputPorts=2
  Scope4 : Scope  Commented=on  NumInputPorts=2
  Scope5 : Scope  Commented=on  NumInputPorts=2
  Scope6 : Scope  Commented=on  NumInputPorts=4
  Signal Builder : Subsystem  Tag=STV Subsys  Commented=on  LoadFcn=sigbuilder_block('load');  StartFcn=sigbuilder_block('start');  StopFcn=sigbuilder_block('stop');  ClipboardFcn=sigbuilder_block('clipboard');  mask(Sigbuilder block){tuvar=[0:10]}
      mask help: Simulink:masks:SigbuilderBlock_MD
      mask init:
      | if ~strcmp(get_param(bdroot(gcbh),'SimulationStatus'),'stopped') tuvar = sigbuilder_block('maskInit'); end
      settings: CopyFcn=sigbuilder_block('copy');  DeleteFcn=sigbuilder_block('delete');  ModelCloseFcn=sigbuilder_block('modelClose');  PreSaveFcn=sigbuilder_block('preSave');  PauseFcn=sigbuilder_block('pause');  ContinueFcn=sigbuilder_block('continue');  NameChangeFcn=sigbuilder_block('namechange');  OpenFcn=sigbuilder_block('open',[5.4 30 1141.2 522.6 ]);  CloseFcn=sigbuilder_block('close');
      mask Display: plot(0, 0, 100, 100,[2, 2, 32, 32, 2], [68, 8, 8, 68, 68],[32, 2], [38, 38], [32, 19, 2],[53, 60, 44], [32, 17, 17, 2],[16, 16, 31, 31]);txt = getActiveGroup(gcbh);text(2, 100, txt,'verticalAlignment', 'top');
  Subtract : Sum
  Switch : Switch  Criteria=u2 > Threshold
  Switch1 : Switch  Criteria=u2 > Threshold
  Terminator{,1..4} (5 alike) : Terminator
  "Torque model 1 -- redacted" : Subsystem  Commented=on
  Vw_mps : Constant  Commented=on  Value=-2
  Zero-Order Hold2 : ZeroOrderHold  SampleTime=-1
  Zero-Order Hold3 : ZeroOrderHold  SampleTime=-1
  acc_deacc_detect : RateLimiter  RisingSlewLimit=1000  FallingSlewLimit=-10e5  SampleTimeMode=inherited
  ad : Derivative
  braking limits kmph1 : Saturate  UpperLimit=0  LowerLimit=-40
  braking rate limiter1 : RateLimiter  RisingSlewLimit=10  FallingSlewLimit=-100  SampleTimeMode=inherited
  break eff.1 : Gain  Gain=-5
  conv2mps1 : Gain  Gain=1/3.6
  conv2mps2 : Gain  Commented=on  Gain=1.65
  eff. coeff : Gain
  enable : Constant
  gradient generation : Subsystem  Tag=STV Subsys  LoadFcn=sigbuilder_block('load');  StartFcn=sigbuilder_block('start');  StopFcn=sigbuilder_block('stop');  ClipboardFcn=sigbuilder_block('clipboard');  mask(Sigbuilder block){tuvar=[0:10]}
      mask help: Simulink:masks:SigbuilderBlock_MD
      mask init:
      | if ~strcmp(get_param(bdroot(gcbh),'SimulationStatus'),'stopped') tuvar = sigbuilder_block('maskInit'); end
      settings: CopyFcn=sigbuilder_block('copy');  DeleteFcn=sigbuilder_block('delete');  ModelCloseFcn=sigbuilder_block('modelClose');  PreSaveFcn=sigbuilder_block('preSave');  PauseFcn=sigbuilder_block('pause');  ContinueFcn=sigbuilder_block('continue');  NameChangeFcn=sigbuilder_block('namechange');  OpenFcn=sigbuilder_block('open',[5.4 30 1141.2 522.6 ]);  CloseFcn=sigbuilder_block('close');
      mask Display: plot(0, 0, 100, 100,[2, 2, 32, 32, 2], [68, 8, 8, 68, 68],[32, 2], [38, 38], [32, 19, 2],[53, 60, 44], [32, 17, 17, 2],[16, 16, 31, 31]);txt = getActiveGroup(gcbh);text(2, 100, txt,'verticalAlignment', 'top');
  if accelerating1 : RelationalOperator  Operator=>  OutDataTypeStr=boolean  RndMeth=Simplest
  if braking1 : RelationalOperator  Operator=<  OutDataTypeStr=boolean  RndMeth=Simplest
  km : Display
  kmph : Gain  Gain=3.6
  m : Display  Commented=on
  m <with slip> : Display  Commented=on
  r : Gain  Commented=on  Gain=0.177
  reverse_ref protection : Saturate  UpperLimit=45  LowerLimit=0
  rho (kg/m^3) : Constant  Value=1.2
  rpm1 : Gain  Gain=60/(2*pi)
  scopes : Subsystem  Commented=on
  slip loss : Gain  Gain=0.9
  tire_radPerSec : Gain  Gain=1/0.117
  uctrig1 : Scope  Commented=on
  vehicle_weight (kg) : Constant  Value=290
  vel_vehicle : Gain  Gain=0.177
  wind profile 2474 : Subsystem  Tag=STV Subsys  LoadFcn=sigbuilder_block('load');  StartFcn=sigbuilder_block('start');  StopFcn=sigbuilder_block('stop');  ClipboardFcn=sigbuilder_block('clipboard');  mask(Sigbuilder block){tuvar=[0:10]}
      mask help: Simulink:masks:SigbuilderBlock_MD
      mask init:
      | if ~strcmp(get_param(bdroot(gcbh),'SimulationStatus'),'stopped') tuvar = sigbuilder_block('maskInit'); end
      settings: CopyFcn=sigbuilder_block('copy');  DeleteFcn=sigbuilder_block('delete');  ModelCloseFcn=sigbuilder_block('modelClose');  PreSaveFcn=sigbuilder_block('preSave');  PauseFcn=sigbuilder_block('pause');  ContinueFcn=sigbuilder_block('continue');  NameChangeFcn=sigbuilder_block('namechange');  OpenFcn=sigbuilder_block('open',[5.4 30 1141.2 522.6 ]);  CloseFcn=sigbuilder_block('close');
      mask Display: plot(0, 0, 100, 100,[2, 2, 32, 32, 2], [68, 8, 8, 68, 68],[32, 2], [38, 38], [32, 19, 2],[53, 60, 44], [32, 17, 17, 2],[16, 16, 31, 31]);txt = getActiveGroup(gcbh);text(2, 100, txt,'verticalAlignment', 'top');
  tag scope: F_losses1=global, UC_trig=global, UC_trig_deacc=global, acc_dec_rate=global, act_wheel_drive_trq=global, ad_detect=global, mech_braking=global, mtr_speed_ref=global, mtr_speed_ref_RPM=global, slope_detect=global, speed_ref=global, vspeed_kmph=global, vspeed_mps=global
  wires:
  GB_ratio/1 -> rpm1/1, [mtr_speed_ref]  "motor_wref(rad/s)"
  Bus Selector/1 -> Gain7/1  "<rotor speed>"
  Bus Selector/2 -> Terminator1/1  "<Rotor angle thetam (rad)>"
  vel_vehicle/1 -> eff. coeff/1
  RPM1/1 -> [tire_rpm]  "tire_rpm"
  kmph/1 -> Saturation3/1
  Gain3/1 -> Add/2
  Add3/1 -> [F_losses1], r/1  "F_losses"
  Saturation4/1 -> Display1/1, [vspeed_mps]  "vehicle_velocity_mps"
  GB_r2w/1 -> RPM1/1, vel_vehicle/1  "tire_radps"
  [Fd] -> Gain8/1
  [speed_ref] -> tire_radPerSec/1  "speed_ref"
  [rotorSens] -> Bus Selector/1
  eff. coeff/1 -> Saturation4/1, kmph/1  "vehicle_speed"
  wind profile 2474/1(Wind_LF) -> [wind_speed]
  r/1 -> Display9/1, Saturation5/1  "T_slope"
  F_drag/1 -> 200Nmax/1  "F_drag"
  tire_radPerSec/1 -> GB_ratio/1
  rho (kg/m^3)/1 -> Mux/1
  rpm1/1 -> [mtr_speed_ref_RPM]
  Saturation3/1 -> [vspeed_kmph], Display/1  "v_kmph"
  Mux1/1 -> Fgx/1, Display4/1, Fgy/1
  gradient generation/2(LF_stable_gradient) -> [gradient]  "gradient"
  Frontal Area m^2/1 -> Mux/4
  Fgx/1 -> Gain1/1  "Fg_x"
  -grad/1 -> Switch/3
  [vspeed_mps] -> Add/1
  Cd/1 -> Mux/3
  From1/1 -> conv2mps2/1
  Add/1 -> Mux/2
  Add1/1 -> Display6/1, [act_wheel_drive_trq]  "act_whl_trq"
  Mux/1 -> F_drag/1
  Fgy/1 -> Terminator2/1
  [wind_speed] -> Gain3/1
  Switch/1 -> [slope_detect]  "grad+-"
  [gradient] -> Switch/2, Saturation/1
  +grad/1 -> Switch/1
  vehicle_weight (kg)/1 -> Mux1/2
  Gain7/1 -> GB_r2w/1
  [speed_user_input] -> Subtract/1  "user_input_speed(m/s)"
  Subtract/1 -> reverse_ref protection/1  "speed_refa"
  [vspeed_mps] -> Scope5/1
  [trq_in2] -> Scope6/4  "torque input 2 alternative"
  [act_wheel_drive_trq] -> Scope6/3  "actual wheel drive torque"
  [vspeed_mps] -> Scope6/1  "speed (m/s)"
  Gain8/1 -> Add3/2
  200Nmax/1 -> Scope5/2, Display3/1, [Fd]  "drag_force"
  [slope_detect] -> Scope4/2
  Gain5/1 -> Subtract/2  "braking_reduction"
  conv2mps1/1 -> braking rate limiter1/1
  [internal_sref] -> Derivative3/1
  [mech_braking] -> Gain5/1
  [gradient] -> Scope4/1
  [torque_input] -> Scope6/2  "Torque input"
  Relational Operator1/1 -> [ad_rel2]
  ad/1 -> Relay2/1
  Derivative5/1 -> Saturation7/1
  Relational Operator4/1 -> Monostable/1
  Constant2/1 -> if accelerating1/2, if braking1/2
  [ad_detect] -> Scope10/4
  [mech_braking] -> Scope10/7
  Relational Operator/1 -> [ad_rel]
  Data Type Conversion3/1 -> Derivative4/1
  Monostable1/1 -> Scope12/3, Scope13/3, [UC_trig_deacc], Monostable2/1  "UC_trig_decel"
  [ad_rel] -> Scope10/3
  [UC_trig] -> Scope12/2
  Saturation7/1 -> uctrig1/1, Relational Operator4/1
  [internal_sref] -> Scope12/1
  acc_deacc_detect/1 -> [acc_dec_rate]  "acc_deacc_rate"
  Constant3/1 -> Relational Operator1/2, Relational Operator/2
  braking rate limiter1/1 -> Scope14/2, [mech_braking]  "mech_braking"
  Data Type Conversion2/1 -> Derivative5/1
  [ad_rel] -> Scope11/2
  Relational Operator5/1 -> Monostable1/1, Scope13/2
  [ad_rel2] -> Scope10/8
  Zero-Order Hold2/1 -> Data Type Conversion2/1
  [ad_rel2] -> Scope11/3
  braking limits kmph1/1 -> conv2mps1/1
  Relay2/1 -> Relational Operator/1, Relational Operator1/1, [A]
  Constant5/1 -> Product3/2
  Monostable2/1 -> break eff.1/1
  Zero-Order Hold3/1 -> Data Type Conversion3/1
  [acc_dec_rate] -> Scope11/1
  Gain9/1 -> Terminator/1
  [UC_trig] -> Scope10/5
  Derivative4/1 -> Saturation8/1
  Monostable/1 -> [UC_trig]  "UC_trig_accel"
  [internal_sref] -> Scope14/1, Scope13/1
  [speed_user_input] -> [internal_sref]
  if accelerating1/1 -> Zero-Order Hold2/1
  Constant4/1 -> Relational Operator5/2, Relational Operator4/2
  Saturation8/1 -> Relational Operator5/1
  Logical Operator/1 -> Product3/1
  Signal Builder/1(Signal 2) -> Gain9/1
  [UC_trig] -> Logical Operator/1
  break eff.1/1 -> Product3/3
  if braking1/1 -> Zero-Order Hold3/1
  [A] -> Scope10/6
  Derivative3/1 -> ad/1, acc_deacc_detect/1, Relay1/1
  Product3/1 -> braking limits kmph1/1
  Relay1/1 -> [ad_detect], if accelerating1/1, if braking1/1  "ad_detect"
  [internal_sref] -> Scope10/1
  [acc_dec_rate] -> Scope10/2
  Saturation5/1 -> Add1/2
  conv2mps2/1 -> Display5/1, Add1/1
  Gain1/1 -> Display2/1, Add3/1  "Fg_x <kg>"
  enable/1 -> Mux1/3
  [gradient] -> Abs1/1
  Abs1/1 -> Switch1/2
  Constant/1 -> Switch1/1
  Constant1/1 -> Switch1/3
  Switch1/1 -> Mux1/4
  Saturation/1 -> Mux1/1
  reverse_ref protection/1 -> [speed_ref]  "speed_ref"
  slip loss/1 -> m <with slip>/1  "m (with slip)"
  Discrete-Time Integrator/1 -> Gain/1, slip loss/1, m/1  "meter"
  Gain/1 -> km/1
  [vspeed_mps] -> Discrete-Time Integrator/1
  gradient generation/1(HF_gradient) -> Terminator3/1
  Gradient generator/1(Gradient) -> Terminator4/1  "gradient"
